simulink subsystem "MultibodySuspensionSSC"  (R2025a)
settings: Solver=VariableStepAuto  StartTime=0.0  StopTime=10.0  RelTol=1e-3
undefined symbols (not defined in the file): EnvGrvty, FrntRef, LAc, LAf, LAr, PlntVehDstCGFrntAxl, PlntVehDstCGRearAxl, PlntVehMass, PlntVehMultiBody, PlntVehMultiBodyGeom, RearRef, StrRodFL, StrRodFR, StrRodRL, StrRodRR, UAc, UAf, UAr, WheelFL, WheelFR, WheelRL, WheelRR, X, Y, Z
libraries: sm_lib x450, fl_lib x96, nesl_utility x64, sdl_lib x8
(part 3 of 17)

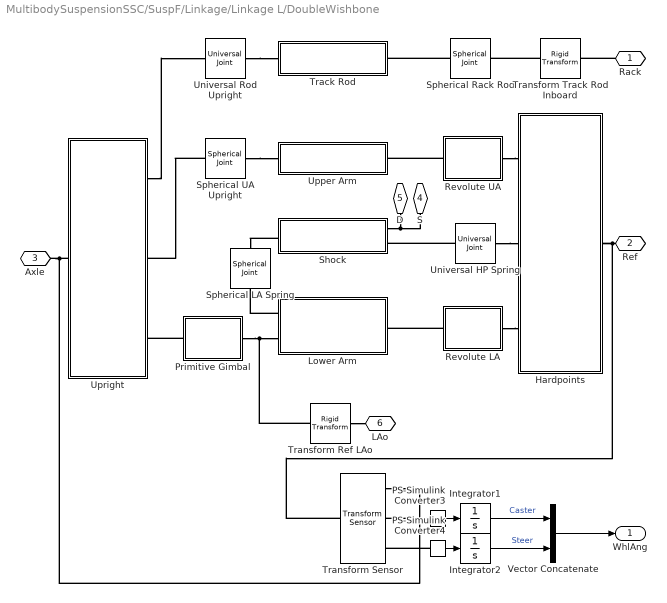
== system MultibodySuspensionSSC/SuspF/Linkage/Linkage L/DoubleWishbone ==
  Hardpoints : Subsystem  mask(Hardpoints, Subframe and Chassis){popup_leftRight=Left, hp_in_f_ua=hp_in_f_ua, hp_in_r_ua=hp_in_r_ua, hp_in_f_la=hp_in_f_la, hp_in_r_la=hp_in_r_la, hp_spr_top=hp_spr_top, clr_hp=clr_hp, opc_hp=opc_hp, size_hp=size_hp}
      mask prompts: popup_leftRight "Left/Right"; hp_in_f_ua "Upper Arm Front [xyz] (m)"; hp_in_r_ua "Upper Arm Rear [xyz] (m)"; hp_in_f_la "Lower Arm Front [xyz] (m)"; hp_in_r_la "Lower Arm Rear [xyz] (m)"; hp_spr_top "Spring [xyz] (m)"
      mask help: Hardpoints for linkage connection points to chassis. Defined relative to an axle reference point.
      mask init:
      | % Set parameter for mirroring (+y or -y)
      | if(popup_leftRight == 1)
      |     rhs_susp = 1;    
      | elseif(popup_leftRight == 2)
      |     rhs_susp = -1;
      | end
      | 
      | rhs_hp = [1 rhs_susp 1];
      | 
      | % Calculate lengths and displacments
      | %len_la_f2r = norm(hp_in_f_la-hp_in_r_la);
      | %len_ua_f2r = norm(hp_in_f_ua-hp_in_r_ua);
      | 
      | % Calculate angle between arm-to-chassis attachment axis
      | % and outboard to inboard front, outboard to inboard rear.
      | % Used to orient z-axis of hardpoint frames along vector 
      | % from inboard points to outboard point.
      | % Angles calculated in World Frame
      | %angle_la_f2r_yaw   =  atan2d(hp_in_f_la(2)-hp_in_r_la(2),hp_in_f_la(1)-hp_in_r_la(1));
      | %angle_la_f2r_pitch = -asind((hp_in_f_la(3)-hp_in_r_la(3))/len_la_f2r);
      | 
      | %angle_ua_f2r_yaw   =  atan2d(hp_in_f_ua(2)-hp_in_r_ua(2),hp_in_f_ua(1)-hp_in_r_ua(1));
      | %angle_ua_f2r_pitch = -asind((hp_in_f_ua(3)-hp_in_r_ua(3))/len_ua_f2r);
      mask TypeOptions popup_leftRight: Left | Right
      mask TypeOptions clr_hp: Subsystem/Vis HP LAf/GraphicDiffuseColor | Vis HP LAr/GraphicDiffuseColor | Vis HP Spring/GraphicDiffuseColor | Vis HP UAf/GraphicDiffuseColor | Vis HP UAr/GraphicDiffuseColor
      mask TypeOptions opc_hp: Subsystem/Vis HP LAf/GraphicOpacity | Vis HP LAr/GraphicOpacity | Vis HP Spring/GraphicOpacity | Vis HP UAf/GraphicOpacity | Vis HP UAr/GraphicOpacity
      mask DialogControl cont_hp Prompt: Hardpoints
      mask DialogControl cont_vis_hp Prompt: Visualization
      mask DialogControl text_clr_hp Prompt: Color [RGB]
      mask DialogControl text_opc_hp Prompt: Opac. (0-1)
      mask DialogControl text_size_hp Prompt: Size (m)
      mask DialogControl text_hp Prompt: Hardpoints
  Integrator1 : Integrator
  Integrator2 : Integrator
  Lower Arm : Subsystem  mask(Lower Arm (Wishbone)){popup_leftRight=Left, hp_in_f=hp_in_f_la, hp_in_r=hp_in_r_la, hp_out=hp_out_la, hp_spr=hp_spr_bot, la_mass=la_mass, clr_la=clr_la, opc_la=opc_la, radius_la=radius_la}
      mask prompts: popup_leftRight "Left/Right"; hp_in_f "Inboard Front [xyz] (m)"; hp_in_r "Inboard Rear [xyz] (m)"; hp_out "Outboard [xyz] (m)"; hp_spr "Spring [xyz] (m)"; la_mass "Mass (kg)"; clr_la "Color [RGB]"; opc_la "Opacity (0-1)"; radius_la "Radius (m)"
      mask help: This subsystem models the lower arm of a wishbone suspension. It can be configured to have one or two attachment points to the chassis. There are connections to the upright and spring.
      mask init:
      | % Set parameter for mirroring (+y or -y)
      | if(popup_leftRight == 1)
      |     rhs_susp = 1;
      | elseif(popup_leftRight == 2)
      |     rhs_susp = -1;
      | end
      | 
      | rhs_hp = [1 rhs_susp 1];
      | 
      | % Calculate lengths and displacments
      | %%%len_front = norm(hp_in_f-hp_out);
      | %%%len_rear  = norm(hp_in_r-hp_out);
      | %%%dist_f2r  = norm(hp_in_f-hp_in_r);
      | 
      | % Vector from outboard hardpoint to spring attachment
      | % Expressed in *World* coordinates
      | %%%xyz_out2spr  = hp_spr-hp_out;
      | 
      | % Calculate angles to align z-axis of arm frames
      | % along vector from inboard points to outboard point
      | % - WORLD FRAME
      | %angle_f2r_pitch = -atan2d(hp_in_f(3)-hp_in_r(3),hp_in_f(1)-hp_in_r(1));
      | %angle_f2r_yaw = atan2d(hp_in_f(2)-hp_in_r(2),hp_in_f(1)-hp_in_r(1));
      | 
      | % Calculate angle between arm-to-chassis attachment axis
      | % and outboard to inboard front, outboard to inboard rear
      | % about axis normal to the arm.
      | % Used to orient z-axis of arm frames along vector 
      | % from inboard points to outboard point
      | %%%angle_f2r_f2out = sm_math_angle_3hp(hp_in_r, hp_in_f, hp_out);
      | %%%angle_r2f_r2out = sm_math_angle_3hp(hp_in_f, hp_in_r, hp_out);
      | 
      | % Obtain angles to reorient frame at outboard hardpoint to global frame
      | % so that outboard to spring attachment calculation can be used
      | % WORLD FRAME - not used
      | %angle_f2r_pitch = sm_math_angle_3hp(hp_in_f.*[1 0 1], hp_in_r.*[1 0 1], [hp_in_f(1) 0 hp_in_r(3)])*sign(hp_in_r(3)-hp_in_f(3))
      | %angle_f2r_yaw = sm_math_angle_3hp(hp_in_f.*[1 1 0], hp_in_r.*[1 1 0], [hp_in_f(1) hp_in_r(2) 0])*sign(hp_in_r(2)-hp_in_f(2))
      | 
      | % Obtain angles to reorient frame at outboard hardpoint to global frame
      | % so that outboard to spring vector in world frame (xyz_out2spr)can be
      | % used. Angles in arm reference frame. 
      | % Same calculation as in hardpoints subsystem.
      | %angle_la_f2r_pitch = -atan2d(hp_in_f(3)-hp_in_r(3),hp_in_f(1)-hp_in_r(1));
      | %angle_la_f2r_yaw   =  atan2d(hp_in_f(2)-hp_in_r(2),hp_in_f(1)-hp_in_r(1));
      | %%%angle_la_f2r_yaw   =  atan2d(hp_in_f(2)-hp_in_r(2),hp_in_f(1)-hp_in_r(1));
      | %%%angle_la_f2r_pitch = -asind((hp_in_f(3)-hp_in_r(3))/dist_f2r);
      | 
      | % -- Calculate rotation of lower arm about joint axis --
      | % Obtain shortest distance from outboard to inboard hardpoint axis
      | % Hypotenuse of triangle for obtaining rotation of arm
      | %%%dist_out2fraxis=len_front*sind(angle_f2r_f2out);
      | 
      | % - Obtain vertical distance of triangle for obtaining rotation of arm
      | % Rotate Inboard Front -> Inboard Rear vector       (r2f)
      | % and Inboard Front -> Outboard vector by yaw angle (r2o)
      | %%%r2f_new = sm_math_rotbasic(hp_in_f'-hp_in_r',-angle_la_f2r_yaw,'z');
      | %%%r2o_new = sm_math_rotbasic(hp_out'-hp_in_r',-angle_la_f2r_yaw,'z');
      | 
      | % Rotate these vectors by pitch angle 
      | %%%r2f_wld = sm_math_rotbasic(r2f_new,-angle_la_f2r_pitch,'y');
      | %%%r2o_wld = sm_math_rotbasic(r2o_new,-angle_la_f2r_pitch,'y');
      | 
      | % Height for angle calculation
      | % After two rotations, can look at z-axis components
      | %%%xangle_height = r2f_wld(3)-r2o_wld(3);
      | 
      | % Calculate angle about f-r axis
      | %%%angle_la_f2raxis = asind(xangle_height/dist_out2fraxis);
      | 
      | % Need additional point to figure out angle with respect to global x-axis
      | % WORLD - Not used
      | %dxpcnt_outfraxis = (hp_out(1)-hp_in_r(1))/(hp_in_f(1)-hp_in_r(1));
      | %hp_rollcalc = hp_in_r+(hp_in_f-hp_in_r)*dxpcnt_outfraxis;
      | %angle_outfr_roll = -sm_math_angle_3hp(hp_rollcalc.*[0 1 1], hp_out.*[0 1 1], [0 hp_rollcalc(2) hp_out(3)])
      | %angle_outfr_roll = -atan2d(hp_out(3)-hp_rollcalc(3),hp_out(2)-hp_rollcalc(2));
      mask Help: web ('sm_car_lower_arm_help.html')
      mask TypeOptions popup_leftRight: Left | Right
      mask TypeOptions clr_la: Arm F/clr_solid | Arm R/clr_solid | Arm Spring/clr_solid
      mask TypeOptions opc_la: Arm F/opc_solid | Arm R/opc_solid | Arm Spring/opc_solid
      mask TypeOptions radius_la: Arm F/rad_solid | Arm R/rad_solid | Arm Spring/rad_solid
      mask DialogControl cont_ua Prompt: LA
      mask DialogControl cont_vis_la Prompt: Visualization
  PS-Simulink Converter3 : nesl_utility/PS-Simulink Converter  PhysicalDomain=network_engine_domain  SubClassName=ps_output  LeftPortType=input  RightPortType=output  PseudoPeriodic=off  Frequencies=[]  VectorFormat=inherit  Unit=inherit  AffineConversion=off
  PS-Simulink Converter4 : nesl_utility/PS-Simulink Converter  PhysicalDomain=network_engine_domain  SubClassName=ps_output  LeftPortType=input  RightPortType=output  PseudoPeriodic=off  Frequencies=[]  VectorFormat=inherit  Unit=inherit  AffineConversion=off
  Primitive Gimbal : Subsystem
      settings: LibrarySourceBlock=sm_car_4post_lib/Suspension and Steering/Linkage/Linkage L/DoubleWishbone/Primitive Gimbal
  Revolute LA : Subsystem  VariantControl=Rigid_1Rev
  Revolute UA : Subsystem  VariantControl=Rigid_1Rev
  Shock : Subsystem  mask(Shock){shock_pist_mass=shock_pist_mass, shock_cyl_mass=shock_cyl_mass, hp_spr_top=hp_spr_top, hp_spr_bot=hp_spr_bot, up_lim_bumpstop=up_lim_bumpstop, low_lim_bumpstop=low_lim_bumpstop, clr_conn_shock=clr_conn_shock, opc_conn_shock=opc_conn_shock, size_conn_shock=size_conn_shock, clr_shock_cyl=clr_shock_cyl, opc_shock_cyl=opc_shock_cyl, radius_shock_cyl=radius_shock_cyl, clr_shock_piston=clr_shock_piston, opc_shock_piston=opc_shock_piston, clr_shock_bumpstop=clr_shock_bumpstop, opc_shock_bumpstop=opc_shock_bumpstop, deadvol_len_shock_cyl=deadvol_len_shock_cyl, piston_len_shock=piston_len_shock, cyl_cap_len_shock=cyl_cap_len_shock, bumpstop_len_shock=bumpstop_len_shock}
      mask prompts: shock_pist_mass "Piston Mass (kg)"; shock_cyl_mass "Cylinder Mass (kg)"; hp_spr_top "Spring Top [xyz] (m)"; hp_spr_bot "Spring Bottom [xyz] (m)"; up_lim_bumpstop "Upper Limit Bumpstop (m)"; low_lim_bumpstop "Lower Limit Bumpstop (m)"; deadvol_len_shock_cyl "Dead Volume Height (m)"; piston_len_shock "Piston Length (m)"; cyl_cap_len_shock "Cylinder Cap Length (m)"; bumpstop_len_shock "Bumpstop Length (m)"
      mask help: Mechanical parts and joint modeling shock absorber.
      mask init:
      | init_spr_len = norm(hp_spr_top-hp_spr_bot);
      | 
      | rod_length = init_spr_len-deadvol_len_shock_cyl-cyl_cap_len_shock-abs(low_lim_bumpstop);
      | 
      | bumpstop_xc_rev = [0 0; 0.5 0; 0.7 1; 0 1].*[radius_shock_cyl bumpstop_len_shock];
      | 
      | cyl_wall_length = piston_len_shock+abs(low_lim_bumpstop)+abs(up_lim_bumpstop)+deadvol_len_shock_cyl;
      mask TypeOptions shock_pist_mass: Piston/Rod/Mass
      mask TypeOptions shock_cyl_mass: Cylinder/Wall/Mass
      mask TypeOptions clr_conn_shock:
      | Vis
      | Spring
      | LA/GraphicDiffuseColor | Vis
      | Spring
      | HP/GraphicDiffuseColor
      mask TypeOptions opc_conn_shock:
      | Vis
      | Spring
      | LA/GraphicOpacity | Vis
      | Spring
      | HP/GraphicOpacity
      mask TypeOptions clr_shock_cyl: Cylinder/Cap Bottom/GraphicDiffuseColor | Cylinder/Cap Top/GraphicDiffuseColor | Cylinder/Wall/GraphicDiffuseColor
      mask TypeOptions clr_shock_piston: Piston/Cap/GraphicDiffuseColor | Piston/Piston/GraphicDiffuseColor | Piston/Rod/GraphicDiffuseColor
      mask TypeOptions opc_shock_piston: Piston/Cap/GraphicOpacity | Piston/Piston/GraphicOpacity | Piston/Rod/GraphicOpacity
      mask TypeOptions clr_shock_bumpstop: Piston/Bumpstop/GraphicDiffuseColor
      mask TypeOptions opc_shock_bumpstop: Piston/Bumpstop/GraphicOpacity
      mask DialogControl cont_shock Prompt: Shock
      mask DialogControl cont_vis_shock Prompt: Visualization
      mask DialogControl text_clr_shock Prompt: Color  [RGB]
      mask DialogControl text_opc_shock Prompt: Opac. (0-1)
      mask DialogControl text_size_shock Prompt: Size (m)
      mask DialogControl text_conn_shock Prompt: Connections
      mask DialogControl text_shock_cyl Prompt: Cylinder
      mask DialogControl text_shock_piston Prompt: Piston
      mask DialogControl text_piston_radius Prompt: <cylinder radius>
      mask DialogControl text_shock_bumpstop Prompt: Bumpstop
      mask DialogControl text_bumpstop_radius Prompt: <cylinder radius>
  Spherical LA Spring : sm_lib/Joints/Spherical Joint  JointMode=Normal  CompositeWrenchDir=FollowerOnBase  CompositeWrenchFrame=BaseFrame  SenseConstraintForce=off  SenseConstraintTorque=off  SenseTotalForce=off  SenseTotalTorque=off  PositionTargetSpecify=off  PositionTargetPriority=High  PositionTargetRotationMethod=None  PositionTargetFollAlignAxisA=+X  PositionTargetBaseAlignAxisA=+Y  PositionTargetFollAlignAxisB=+Y  PositionTargetBaseAlignAxisB=+Z  PositionTargetRotationStandardAxis=+Z  PositionTargetRotationAngle=0.0  PositionTargetRotationAngleUnits=deg  PositionTargetRotationArbitraryAxis=[0 0 1]  PositionTargetRotationSequenceAxes=FollowerAxes  PositionTargetRotationSequence=XYX  PositionTargetRotationSequenceAngles=[0 0 0]  PositionTargetRotationSequenceAnglesUnits=deg  PositionTargetRotationMatrix=[1 0 0; 0 1 0; 0 0 1]  PositionTargetQuaternion=[1 0 0 0]  VelocityTargetSpecify=off  VelocityTargetPriority=High  VelocityTargetValue=[0 0 0]  VelocityTargetValueUnits=deg/s  VelocityTargetInFollowerFrame=on  EqPosRotationMethod=None  EqPosFollAlignAxisA=+X  EqPosBaseAlignAxisA=+Y  EqPosFollAlignAxisB=+Y  EqPosBaseAlignAxisB=+Z  EqPosRotationStandardAxis=+Z  EqPosRotationAngle=0.0  EqPosRotationAngleUnits=deg  EqPosRotationArbitraryAxis=[0 0 1]  EqPosRotationSequenceAxes=FollowerAxes  EqPosRotationSequence=XYX  EqPosRotationSequenceAngles=[0 0 0]  EqPosRotationSequenceAnglesUnits=deg  EqPosRotationMatrix=[1 0 0; 0 1 0; 0 0 1]  EqPosQuaternion=[1 0 0 0]  SpringStiffness=0  SpringStiffnessUnits=N*m/deg  DampingCoefficient=0  DampingCoefficientUnits=N*m/(deg/s)  LowerLimitSpecify=off  LowerLimitBound=15  LowerLimitBoundUnits=deg  LowerLimitStiffness=1e4  LowerLimitStiffnessUnits=N*m/deg  LowerLimitDamping=10  LowerLimitDampingUnits=N*m/(deg/s)  LowerLimitTransitionRegionWidth=0.1  LowerLimitTransitionRegionWidthUnits=deg  UpperLimitSpecify=off  UpperLimitBound=45  UpperLimitBoundUnits=deg  UpperLimitStiffness=1e4  UpperLimitStiffnessUnits=N*m/deg  UpperLimitDamping=10  UpperLimitDampingUnits=N*m/(deg/s)  UpperLimitTransitionRegionWidth=0.1  UpperLimitTransitionRegionWidthUnits=deg  TorqueActuationMode=NoTorque  ActuateTorqueX=off  ActuateTorqueY=off  ActuateTorqueZ=off  ActuateTorque=off  ActuationFrame=BaseFrame  SensePosition=off  SenseVelocityX=off  SenseVelocityY=off  SenseVelocityZ=off  SenseVelocity=off  SenseAccelerationX=off  SenseAccelerationY=off  SenseAccelerationZ=off  SenseAcceleration=off  SenseLowerLimitTorqueMag=off  SenseUpperLimitTorqueMag=off  SensingFrame=BaseFrame
      settings: LibrarySourceBlock=|
      | sm_car_4post_lib/Suspension and Steering/Linkage/Linkage L/DoubleWishbone/Spherical
      | LA Spring
  Spherical Rack Rod : sm_lib/Joints/Spherical Joint  JointMode=Normal  CompositeWrenchDir=FollowerOnBase  CompositeWrenchFrame=BaseFrame  SenseConstraintForce=off  SenseConstraintTorque=off  SenseTotalForce=off  SenseTotalTorque=off  PositionTargetSpecify=off  PositionTargetPriority=High  PositionTargetRotationMethod=None  PositionTargetFollAlignAxisA=+X  PositionTargetBaseAlignAxisA=+Y  PositionTargetFollAlignAxisB=+Y  PositionTargetBaseAlignAxisB=+Z  PositionTargetRotationStandardAxis=+Z  PositionTargetRotationAngle=0.0  PositionTargetRotationAngleUnits=deg  PositionTargetRotationArbitraryAxis=[0 0 1]  PositionTargetRotationSequenceAxes=FollowerAxes  PositionTargetRotationSequence=XYX  PositionTargetRotationSequenceAngles=[0 0 0]  PositionTargetRotationSequenceAnglesUnits=deg  PositionTargetRotationMatrix=[1 0 0; 0 1 0; 0 0 1]  PositionTargetQuaternion=[1 0 0 0]  VelocityTargetSpecify=off  VelocityTargetPriority=High  VelocityTargetValue=[0 0 0]  VelocityTargetValueUnits=deg/s  VelocityTargetInFollowerFrame=on  EqPosRotationMethod=None  EqPosFollAlignAxisA=+X  EqPosBaseAlignAxisA=+Y  EqPosFollAlignAxisB=+Y  EqPosBaseAlignAxisB=+Z  EqPosRotationStandardAxis=+Z  EqPosRotationAngle=0.0  EqPosRotationAngleUnits=deg  EqPosRotationArbitraryAxis=[0 0 1]  EqPosRotationSequenceAxes=FollowerAxes  EqPosRotationSequence=XYX  EqPosRotationSequenceAngles=[0 0 0]  EqPosRotationSequenceAnglesUnits=deg  EqPosRotationMatrix=[1 0 0; 0 1 0; 0 0 1]  EqPosQuaternion=[1 0 0 0]  SpringStiffness=0  SpringStiffnessUnits=N*m/deg  DampingCoefficient=0  DampingCoefficientUnits=N*m/(deg/s)  LowerLimitSpecify=off  LowerLimitBound=15  LowerLimitBoundUnits=deg  LowerLimitStiffness=1e4  LowerLimitStiffnessUnits=N*m/deg  LowerLimitDamping=10  LowerLimitDampingUnits=N*m/(deg/s)  LowerLimitTransitionRegionWidth=0.1  LowerLimitTransitionRegionWidthUnits=deg  UpperLimitSpecify=off  UpperLimitBound=45  UpperLimitBoundUnits=deg  UpperLimitStiffness=1e4  UpperLimitStiffnessUnits=N*m/deg  UpperLimitDamping=10  UpperLimitDampingUnits=N*m/(deg/s)  UpperLimitTransitionRegionWidth=0.1  UpperLimitTransitionRegionWidthUnits=deg  TorqueActuationMode=NoTorque  ActuateTorqueX=off  ActuateTorqueY=off  ActuateTorqueZ=off  ActuateTorque=off  ActuationFrame=BaseFrame  SensePosition=off  SenseVelocityX=off  SenseVelocityY=off  SenseVelocityZ=off  SenseVelocity=off  SenseAccelerationX=off  SenseAccelerationY=off  SenseAccelerationZ=off  SenseAcceleration=off  SenseLowerLimitTorqueMag=off  SenseUpperLimitTorqueMag=off  SensingFrame=BaseFrame
      settings: LibrarySourceBlock=|
      | sm_car_4post_lib/Suspension and Steering/Linkage/Linkage L/DoubleWishbone/Spherical
      | Rack Rod
  Spherical UA Upright : sm_lib/Joints/Spherical Joint  JointMode=Normal  CompositeWrenchDir=FollowerOnBase  CompositeWrenchFrame=BaseFrame  SenseConstraintForce=off  SenseConstraintTorque=off  SenseTotalForce=off  SenseTotalTorque=off  PositionTargetSpecify=on  PositionTargetPriority=High  PositionTargetRotationMethod=StandardAxis  PositionTargetFollAlignAxisA=+X  PositionTargetBaseAlignAxisA=+Y  PositionTargetFollAlignAxisB=+Y  PositionTargetBaseAlignAxisB=+Z  PositionTargetRotationStandardAxis=+Z  PositionTargetRotationAngle=0.0  PositionTargetRotationAngleUnits=deg  PositionTargetRotationArbitraryAxis=[0 0 1]  PositionTargetRotationSequenceAxes=FollowerAxes  PositionTargetRotationSequence=XYX  PositionTargetRotationSequenceAngles=[0 0 0]  PositionTargetRotationSequenceAnglesUnits=deg  PositionTargetRotationMatrix=[1 0 0; 0 1 0; 0 0 1]  PositionTargetQuaternion=[1 0 0 0]  VelocityTargetSpecify=off  VelocityTargetPriority=High  VelocityTargetValue=[0 0 0]  VelocityTargetValueUnits=deg/s  VelocityTargetInFollowerFrame=on  EqPosRotationMethod=None  EqPosFollAlignAxisA=+X  EqPosBaseAlignAxisA=+Y  EqPosFollAlignAxisB=+Y  EqPosBaseAlignAxisB=+Z  EqPosRotationStandardAxis=+Z  EqPosRotationAngle=0.0  EqPosRotationAngleUnits=deg  EqPosRotationArbitraryAxis=[0 0 1]  EqPosRotationSequenceAxes=FollowerAxes  EqPosRotationSequence=XYX  EqPosRotationSequenceAngles=[0 0 0]  EqPosRotationSequenceAnglesUnits=deg  EqPosRotationMatrix=[1 0 0; 0 1 0; 0 0 1]  EqPosQuaternion=[1 0 0 0]  SpringStiffness=0  SpringStiffnessUnits=N*m/deg  DampingCoefficient=0  DampingCoefficientUnits=N*m/(deg/s)  LowerLimitSpecify=off  LowerLimitBound=15  LowerLimitBoundUnits=deg  LowerLimitStiffness=1e4  LowerLimitStiffnessUnits=N*m/deg  LowerLimitDamping=10  LowerLimitDampingUnits=N*m/(deg/s)  LowerLimitTransitionRegionWidth=0.1  LowerLimitTransitionRegionWidthUnits=deg  UpperLimitSpecify=off  UpperLimitBound=45  UpperLimitBoundUnits=deg  UpperLimitStiffness=1e4  UpperLimitStiffnessUnits=N*m/deg  UpperLimitDamping=10  UpperLimitDampingUnits=N*m/(deg/s)  UpperLimitTransitionRegionWidth=0.1  UpperLimitTransitionRegionWidthUnits=deg  TorqueActuationMode=NoTorque  ActuateTorqueX=off  ActuateTorqueY=off  ActuateTorqueZ=off  ActuateTorque=off  ActuationFrame=BaseFrame  SensePosition=off  SenseVelocityX=off  SenseVelocityY=off  SenseVelocityZ=off  SenseVelocity=off  SenseAccelerationX=off  SenseAccelerationY=off  SenseAccelerationZ=off  SenseAcceleration=off  SenseLowerLimitTorqueMag=off  SenseUpperLimitTorqueMag=off  SensingFrame=BaseFrame
      settings: LibrarySourceBlock=|
      | sm_car_4post_lib/Suspension and Steering/Linkage/Linkage L/DoubleWishbone/Spherical
      | UA Upright
  Track Rod : Subsystem  VariantControl=Steer  mask{popup_leftRight=Left, hp_in=hp_in_rod, hp_out=hp_upr_rod, rod_mass=rod_mass, clr_conn_rod=clr_conn_rod, opc_conn_rod=opc_conn_rod, size_conn_rod=size_conn_rod, clr_rod=clr_rod, opc_rod=opc_rod, radius_rod=radius_rod}
      mask prompts: popup_leftRight "Left/Right"; hp_in "Inboard [xyz] (m)"; hp_out "Outboard [xyz] (m)"; rod_mass "Mass (kg)"; clr_rod "Color [RGB]"; opc_rod "Opacity (0-1)"; radius_rod "Radius (m)"
      mask init:
      | if(popup_leftRight == 1)
      |     rhs_rod = 1;
      | elseif(popup_leftRight == 2)
      |     rhs_rod = -1;
      | end
      | 
      | % Calculate lengths
      | %%%rod_len = norm(hp_out-hp_in);
      mask TypeOptions popup_leftRight: Left | Right
      mask TypeOptions rod_mass: Rod/Mass
      mask TypeOptions clr_conn_rod:
      | Vis
      | Upright
      | Steer/GraphicDiffuseColor | Vis
      | Rack
      | Rod/GraphicDiffuseColor
      mask TypeOptions opc_conn_rod:
      | Vis
      | Upright
      | Steer/GraphicOpacity | Vis
      | Rack
      | Rod/GraphicOpacity
      mask TypeOptions clr_rod: Rod/clr_solid
      mask TypeOptions opc_rod: Rod/opc_solid
      mask TypeOptions radius_rod: Rod/rad_solid
      mask DialogControl cont_rod Prompt: Rod
      mask DialogControl grp_rod Prompt: Rod
      mask DialogControl cont_vis_rod Prompt: Visualization
      mask DialogControl text_clr_rod Prompt: Color [RGB]
      mask DialogControl text_opc_rod Prompt: Opac. (0-1)
      mask DialogControl text_size_rod Prompt: Size (m)
      mask DialogControl text_conn_rod Prompt: Connections
      mask DialogControl text_rod_rod Prompt: Rod
  Transform Ref LAo : sm_lib/Frames and Transforms/Rigid Transform  RotationMethod=None  FollAlignAxisA=+X  BaseAlignAxisA=+Y  FollAlignAxisB=+Y  BaseAlignAxisB=+Z  RotationStandardAxis=+Z  RotationAngle=0.0  RotationAngleUnits=deg  RotationArbitraryAxis=[0 0 1]  RotationSequenceAxes=FollowerAxes  RotationSequence=XYX  RotationSequenceAngles=[0 0 0]  RotationSequenceAnglesUnits=deg  RotationMatrix=[1 0 0; 0 1 0; 0 0 1]  Quaternion=[1 0 0 0]  TranslationMethod=Cartesian  TranslationCartesianOffset=hp_out_la.*[1 rhs_susp 1]  TranslationCartesianOffsetUnits=m  TranslationStandardAxis=+Z  TranslationStandardOffset=0  TranslationStandardOffsetUnits=m  TranslationROffset=0  TranslationROffsetUnits=m  TranslationThetaOffset=0  TranslationThetaOffsetUnits=deg  TranslationZOffset=0  TranslationZOffsetUnits=m
  Transform Sensor : sm_lib/Frames and Transforms/Transform Sensor  MeasurementFrame=NonRotatingBase  RotationSequence=XYX  SenseAngle=off  SenseAxis=off  SenseQ=off  SenseR=off  SenseRotationSequence=off  SenseOmegaX=off  SenseOmegaY=on  SenseOmegaZ=on  SenseOmega=off  SenseQDot=off  SenseRDot=off  SenseRotationSequenceDot=off  SenseAlphaX=off  SenseAlphaY=off  SenseAlphaZ=off  SenseAlpha=off  SenseQDDot=off  SenseRDDot=off  SenseX=off  SenseY=off  SenseZ=off  SenseXYZ=off  SenseRad=off  SenseAzim=off  SenseDist=off  SenseInc=off  SenseXDot=off  SenseYDot=off  SenseZDot=off  SenseXYZDot=off  SenseRadDot=off  SenseAzimDot=off  SenseDistDot=off  SenseIncDot=off  SenseXDDot=off  SenseYDDot=off  SenseZDDot=off  SenseXYZDDot=off  SenseRadDDot=off  SenseAzimDDot=off  SenseDistDDot=off  SenseIncDDot=off
  Transform Track Rod Inboard : sm_lib/Frames and Transforms/Rigid Transform  RotationMethod=None  FollAlignAxisA=+X  BaseAlignAxisA=+Y  FollAlignAxisB=+Y  BaseAlignAxisB=+Z  RotationStandardAxis=+Z  RotationAngle=0.0  RotationAngleUnits=deg  RotationArbitraryAxis=[0 0 1]  RotationSequenceAxes=FollowerAxes  RotationSequence=XYX  RotationSequenceAngles=[0 0 0]  RotationSequenceAnglesUnits=deg  RotationMatrix=[1 0 0; 0 1 0; 0 0 1]  Quaternion=[1 0 0 0]  TranslationMethod=Cartesian  TranslationCartesianOffset=hp_in_rod.*[1 rhs_susp 1]  TranslationCartesianOffsetUnits=m  TranslationStandardAxis=+Z  TranslationStandardOffset=0  TranslationStandardOffsetUnits=m  TranslationROffset=0  TranslationROffsetUnits=m  TranslationThetaOffset=0  TranslationThetaOffsetUnits=deg  TranslationZOffset=0  TranslationZOffsetUnits=m
      settings: LibrarySourceBlock=|
      | sm_car_4post_lib/Suspension and Steering/Linkage/Linkage L/DoubleWishbone/Transform
      | Track Rod Inboard
  Universal HP Spring : sm_lib/Joints/Universal Joint  JointMode=Normal  CompositeWrenchDir=FollowerOnBase  CompositeWrenchFrame=BaseFrame  SenseConstraintForce=off  SenseConstraintTorque=off  SenseTotalForce=off  SenseTotalTorque=off  RxPositionTargetSpecify=off  RxPositionTargetPriority=High  RxPositionTargetValue=0  RxPositionTargetValueUnits=deg  RxVelocityTargetSpecify=off  RxVelocityTargetPriority=High  RxVelocityTargetValue=0  RxVelocityTargetValueUnits=deg/s  RxEquilibriumPosition=0  RxEquilibriumPositionUnits=deg  RxSpringStiffness=0  RxSpringStiffnessUnits=N*m/deg  RxDampingCoefficient=0  RxDampingCoefficientUnits=N*m/(deg/s)  RxLowerLimitSpecify=off  RxLowerLimitBound=-90  RxLowerLimitBoundUnits=deg  RxLowerLimitStiffness=1e4  RxLowerLimitStiffnessUnits=N*m/deg  RxLowerLimitDamping=10  RxLowerLimitDampingUnits=N*m/(deg/s)  RxLowerLimitTransitionRegionWidth=0.1  RxLowerLimitTransitionRegionWidthUnits=deg  RxUpperLimitSpecify=off  RxUpperLimitBound=90  RxUpperLimitBoundUnits=deg  RxUpperLimitStiffness=1e4  RxUpperLimitStiffnessUnits=N*m/deg  RxUpperLimitDamping=10  RxUpperLimitDampingUnits=N*m/(deg/s)  RxUpperLimitTransitionRegionWidth=0.1  RxUpperLimitTransitionRegionWidthUnits=deg  RxTorqueActuationMode=NoTorque  RxMotionActuationMode=ComputedMotion  RxSensePosition=off  RxSenseVelocity=off  RxSenseAcceleration=off  RxSenseTorqueForce=off  RxSenseLowerLimitTorqueForce=off  RxSenseUpperLimitTorqueForce=off  RyPositionTargetSpecify=off  RyPositionTargetPriority=High  RyPositionTargetValue=0  RyPositionTargetValueUnits=deg  RyVelocityTargetSpecify=off  RyVelocityTargetPriority=High  RyVelocityTargetValue=0  RyVelocityTargetValueUnits=deg/s  RyEquilibriumPosition=0  RyEquilibriumPositionUnits=deg  RySpringStiffness=0  RySpringStiffnessUnits=N*m/deg  RyDampingCoefficient=0  RyDampingCoefficientUnits=N*m/(deg/s)  RyLowerLimitSpecify=off  RyLowerLimitBound=-90  RyLowerLimitBoundUnits=deg  RyLowerLimitStiffness=1e4  RyLowerLimitStiffnessUnits=N*m/deg  RyLowerLimitDamping=10  RyLowerLimitDampingUnits=N*m/(deg/s)  RyLowerLimitTransitionRegionWidth=0.1  RyLowerLimitTransitionRegionWidthUnits=deg  RyUpperLimitSpecify=off  RyUpperLimitBound=90  RyUpperLimitBoundUnits=deg  RyUpperLimitStiffness=1e4  RyUpperLimitStiffnessUnits=N*m/deg  RyUpperLimitDamping=10  RyUpperLimitDampingUnits=N*m/(deg/s)  RyUpperLimitTransitionRegionWidth=0.1  RyUpperLimitTransitionRegionWidthUnits=deg  RyTorqueActuationMode=NoTorque  RyMotionActuationMode=ComputedMotion  RySensePosition=off  RySenseVelocity=off  RySenseAcceleration=off  RySenseTorqueForce=off  RySenseLowerLimitTorqueForce=off  RySenseUpperLimitTorqueForce=off
      settings: LibrarySourceBlock=|
      | sm_car_4post_lib/Suspension and Steering/Linkage/Linkage L/DoubleWishbone/Universal
      | HP Spring
  Universal Rod Upright : sm_lib/Joints/Universal Joint  JointMode=Normal  CompositeWrenchDir=FollowerOnBase  CompositeWrenchFrame=BaseFrame  SenseConstraintForce=off  SenseConstraintTorque=off  SenseTotalForce=off  SenseTotalTorque=off  RxPositionTargetSpecify=off  RxPositionTargetPriority=Low  RxPositionTargetValue=0  RxPositionTargetValueUnits=deg  RxVelocityTargetSpecify=off  RxVelocityTargetPriority=High  RxVelocityTargetValue=0  RxVelocityTargetValueUnits=deg/s  RxEquilibriumPosition=0  RxEquilibriumPositionUnits=deg  RxSpringStiffness=0  RxSpringStiffnessUnits=N*m/deg  RxDampingCoefficient=0  RxDampingCoefficientUnits=N*m/(deg/s)  RxLowerLimitSpecify=off  RxLowerLimitBound=-90  RxLowerLimitBoundUnits=deg  RxLowerLimitStiffness=1e4  RxLowerLimitStiffnessUnits=N*m/deg  RxLowerLimitDamping=10  RxLowerLimitDampingUnits=N*m/(deg/s)  RxLowerLimitTransitionRegionWidth=0.1  RxLowerLimitTransitionRegionWidthUnits=deg  RxUpperLimitSpecify=off  RxUpperLimitBound=90  RxUpperLimitBoundUnits=deg  RxUpperLimitStiffness=1e4  RxUpperLimitStiffnessUnits=N*m/deg  RxUpperLimitDamping=10  RxUpperLimitDampingUnits=N*m/(deg/s)  RxUpperLimitTransitionRegionWidth=0.1  RxUpperLimitTransitionRegionWidthUnits=deg  RxTorqueActuationMode=NoTorque  RxMotionActuationMode=ComputedMotion  RxSensePosition=off  RxSenseVelocity=off  RxSenseAcceleration=off  RxSenseTorqueForce=off  RxSenseLowerLimitTorqueForce=off  RxSenseUpperLimitTorqueForce=off  RyPositionTargetSpecify=off  RyPositionTargetPriority=High  RyPositionTargetValue=0  RyPositionTargetValueUnits=deg  RyVelocityTargetSpecify=off  RyVelocityTargetPriority=High  RyVelocityTargetValue=0  RyVelocityTargetValueUnits=deg/s  RyEquilibriumPosition=0  RyEquilibriumPositionUnits=deg  RySpringStiffness=0  RySpringStiffnessUnits=N*m/deg  RyDampingCoefficient=0  RyDampingCoefficientUnits=N*m/(deg/s)  RyLowerLimitSpecify=off  RyLowerLimitBound=-90  RyLowerLimitBoundUnits=deg  RyLowerLimitStiffness=1e4  RyLowerLimitStiffnessUnits=N*m/deg  RyLowerLimitDamping=10  RyLowerLimitDampingUnits=N*m/(deg/s)  RyLowerLimitTransitionRegionWidth=0.1  RyLowerLimitTransitionRegionWidthUnits=deg  RyUpperLimitSpecify=off  RyUpperLimitBound=90  RyUpperLimitBoundUnits=deg  RyUpperLimitStiffness=1e4  RyUpperLimitStiffnessUnits=N*m/deg  RyUpperLimitDamping=10  RyUpperLimitDampingUnits=N*m/(deg/s)  RyUpperLimitTransitionRegionWidth=0.1  RyUpperLimitTransitionRegionWidthUnits=deg  RyTorqueActuationMode=NoTorque  RyMotionActuationMode=ComputedMotion  RySensePosition=off  RySenseVelocity=off  RySenseAcceleration=off  RySenseTorqueForce=off  RySenseLowerLimitTorqueForce=off  RySenseUpperLimitTorqueForce=off
      settings: LibrarySourceBlock=|
      | sm_car_4post_lib/Suspension and Steering/Linkage/Linkage L/DoubleWishbone/Universal
      | Rod Upright
  Upper Arm : Subsystem  mask{popup_leftRight=Left, hp_in_f=hp_in_f_ua, hp_in_r=hp_in_r_ua, hp_out=hp_out_ua, ua_mass=ua_mass, clr_ua=clr_ua, opc_ua=opc_ua, radius_ua=radius_ua}
      mask prompts: popup_leftRight "Left/Right"; hp_in_f "Inboard Front [xyz] (m)"; hp_in_r "Inboard Rear [xyz] (m)"; hp_out "Outboard [xyz] (m)"; ua_mass "Mass (kg)"; clr_ua "Color [RGB]"; opc_ua "Opacity (0-1)"; radius_ua "Radius (m)"
      mask init:
      | if(popup_leftRight == 1)
      |     rhs_susp = 1;
      | elseif(popup_leftRight == 2)
      |     rhs_susp = -1;
      | end
      | 
      | rhs_hp = [1 rhs_susp 1];
      | 
      | % Calculate lengths and displacments
      | %%%len_front = norm(hp_in_f-hp_out);
      | %%%len_rear  = norm(hp_in_r-hp_out);
      | %%%dist_f2r  = norm(hp_in_f-hp_in_r);
      | 
      | % Calculate angle between arm-to-chassis attachment axis
      | % and outboard hard point at each chassis attachment point
      | %%%angle_f2r_f2out = sm_math_angle_3hp(hp_in_r, hp_in_f, hp_out);
      | %%%angle_r2f_r2out = sm_math_angle_3hp(hp_in_f, hp_in_r, hp_out);
      mask TypeOptions popup_leftRight: Left | Right
      mask TypeOptions clr_ua: Arm F/clr_solid | Arm R/clr_solid
      mask TypeOptions opc_ua: Arm F/opc_solid | Arm R/opc_solid
      mask TypeOptions radius_ua: Arm F/rad_solid | Arm R/rad_solid
      mask DialogControl cont_ua Prompt: UA
      mask DialogControl cont_vis_ua Prompt: Visualization
  Upright : Subsystem  mask(Upright){popup_leftRight=Left, hp_ua_out=hp_out_ua, hp_la_out=hp_out_la, hp_upr_cg=hp_upr_cg, hp_upr_wc=hp_upr_wc, hp_upr_rod=hp_upr_rod, atoe=atoe, acamber=acamber, upr_mass=upr_mass, whl_init_spd=whl_init_spd_lr(whlind), clr_conn_upr=clr_conn_upr, opc_conn_upr=opc_conn_upr, size_conn_upr=size_conn_upr, clr_upr=clr_upr, opc_upr=opc_upr, radius_upr=radius_upr, clr_stub_axle=clr_stub_axle, opc_stub_axle=opc_stub_axle, radius_stub_axle=radius_stub_axle}
      mask prompts: popup_leftRight "Left/Right"; hp_ua_out "Upper Arm Outboard [xyz] (m)"; hp_la_out "Lower Arm Outboard [xyz] (m)"; hp_upr_cg "Center of Mass [xyz] (m)"; hp_upr_wc "Wheel Center [xyz] (m)"; hp_upr_rod "Track Rod Outboard [xyz] (m)"; atoe "Toe Angle (deg)"; acamber "Camber Angle (deg)"; upr_mass "Upright Mass (kg)"; whl_init_spd "Initial Wheel Speed (rad/s)"
      mask help: Suspension linkage that holds wheel bearing.
      mask init:
      | % Set parameter for mirroring (+y or -y)
      | if(popup_leftRight == 1)
      |     rhs_upr = 1;
      | elseif(popup_leftRight == 2)
      |     rhs_upr = -1;
      | end
      | rhs_hp = [1 rhs_upr 1];
      | 
      | % Additional hardpoint at center of upright
      | % Used as attachment points for axle and steering arm
      | hp_upr_ctr = (hp_ua_out+hp_la_out)/2;
      | 
      | % Calculate lengths and displacments
      | %%%len_upr  = norm(hp_la_out-hp_ua_out);
      | len_axle = norm(hp_upr_wc-hp_upr_ctr);
      | %%%len_sarm = norm(hp_upr_rod-hp_upr_ctr);
      | %%%len_cg   = norm(hp_upr_cg-hp_upr_ctr);
      | 
      | % Get angle between steering arm and axle about axis perpendicular to upright z-axis
      | %%%angle_axle2upr_perp = sm_math_angle_3hp(hp_ua_out,hp_upr_ctr,hp_upr_wc);
      | %%%angle_rod2upr_perp = sm_math_angle_3hp(hp_ua_out,hp_upr_ctr,hp_upr_rod);
      | %%%angle_cg2upr_perp = sm_math_angle_3hp(hp_ua_out,hp_upr_ctr,hp_upr_cg);
      | 
      | % Get vectors for axle, arm, and cg relative to upright center
      | %%%vec_upr2rod = hp_upr_rod-hp_upr_ctr;
      | %%%vec_upr2wc  = hp_upr_wc-hp_upr_ctr;
      | %%%vec_upr2cg  = hp_upr_cg-hp_upr_ctr;
      | 
      | % Get angles to rotate upright back to World orientation
      | % Two rotations in sequence, first about x then about y
      | %%%angle_x = -90+atan2d(hp_ua_out(3)-hp_la_out(3),hp_ua_out(2)-hp_la_out(2));
      | %%%angle_y = acosd(sqrt((hp_ua_out(3)-hp_la_out(3))^2+(hp_ua_out(2)-hp_la_out(2))^2)/len_upr);
      | 
      | % Rotate vectors for axle, arm, and cg relative to upright center by these angles
      | %%%vec_upr2rod_inUpr1 = sm_math_rotbasic(vec_upr2rod',-angle_x,'x');
      | %%%vec_upr2rod_inUpr = sm_math_rotbasic(vec_upr2rod_inUpr1,angle_y,'y');
      | 
      | %%%vec_upr2wc_inUpr1  = sm_math_rotbasic(vec_upr2wc',-angle_x,'x');
      | %%%vec_upr2wc_inUpr = sm_math_rotbasic(vec_upr2wc_inUpr1,angle_y,'y');
      | 
      | %%%vec_upr2cg_inUpr1  = sm_math_rotbasic(vec_upr2cg',-angle_x,'x');
      | %%%vec_upr2cg_inUpr = sm_math_rotbasic(vec_upr2cg_inUpr1,angle_y,'y');
      | 
      | % Get angle to steering arm and to axle about upright axis
      | %%%angle_rod2upraxis = atan2d(vec_upr2rod_inUpr(2),vec_upr2rod_inUpr(1));
      | %%%angle_wc2upraxis  = atan2d(vec_upr2wc_inUpr(2),vec_upr2wc_inUpr(1));
      | %%%angle_cg2upraxis  = atan2d(vec_upr2cg_inUpr(2),vec_upr2cg_inUpr(1));
      mask TypeOptions popup_leftRight: Left | Right
      mask TypeOptions upr_mass:
      | Inertia
      | CG/Mass
      mask TypeOptions whl_init_spd: Revolute/Revolute/VelocityTargetValue
      mask TypeOptions clr_conn_upr: Vis Upright LA/GraphicDiffuseColor | Vis Upright UA/GraphicDiffuseColor | Vis Wheel Center/GraphicDiffuseColor
      mask TypeOptions opc_conn_upr: Vis Upright LA/GraphicOpacity | Vis Upright UA/GraphicOpacity | Vis Wheel Center/GraphicOpacity
      mask TypeOptions clr_upr: Upright/clr_solid | Steering Arm/clr_solid
      mask TypeOptions opc_upr: Upright/opc_solid | Steering Arm/opc_solid
      mask TypeOptions radius_upr: Upright/rad_solid | Steering Arm/rad_solid
      mask TypeOptions clr_stub_axle: Axle/GraphicDiffuseColor
      mask TypeOptions opc_stub_axle: Axle/GraphicOpacity
      mask TypeOptions radius_stub_axle: Axle/CylinderRadius
      mask DialogControl cont_upright Prompt: Upright
      mask DialogControl grp_init Prompt: Initialization
      mask DialogControl cont_vis_upr Prompt: Visualization
      mask DialogControl text_clr_upr Prompt: Color [RGB]
      mask DialogControl text_opc_upr Prompt: Opac. (0-1)
      mask DialogControl text_size_upr Prompt: Size (m)
      mask DialogControl text_conn_upr Prompt: Connections
      mask DialogControl text_upright Prompt: Upright
      mask DialogControl text_stub_axle Prompt: Stub Axle
  Vector Concatenate : Concatenate
  Rack : PMIOPort  Side=Right
  Ref : PMIOPort  Port=2  Side=Right
  Axle : PMIOPort  Port=3  Side=Left
  S : PMIOPort  Port=4  Side=Left
  D : PMIOPort  Port=5  Side=Left
  LAo : PMIOPort  Port=6  Side=Left
  WhlAng : Outport
  wires:
  Vector Concatenate/1 -> WhlAng/1
  PS-Simulink Converter3/1 -> Integrator1/1
  Integrator1/1 -> Vector Concatenate/1  "Caster"
  PS-Simulink Converter4/1 -> Integrator2/1
  Integrator2/1 -> Vector Concatenate/2  "Steer"
  connections:
  Transform Track Rod Inboard/RConn1 -- Spherical Rack Rod/LConn1
  Spherical Rack Rod/RConn1 -- Track Rod/RConn1
  Universal Rod Upright/LConn1 -- Track Rod/LConn1
  Spherical UA Upright/RConn1 -- Upright/RConn2
  Primitive Gimbal/LConn1 -- Transform Ref LAo/RConn1 -- Lower Arm/LConn2
  Revolute LA/RConn1 -- Lower Arm/RConn1
  Spherical UA Upright/LConn1 -- Upper Arm/LConn1
  Primitive Gimbal/RConn1 -- Upright/RConn3
  Lower Arm/LConn1 -- Spherical LA Spring/LConn1
  Revolute LA/LConn1 -- Hardpoints/LConn3
  Revolute UA/RConn1 -- Upper Arm/RConn1
  D/RConn1 -- S/RConn1 -- Shock/RConn1
  Rack/RConn1 -- Transform Track Rod Inboard/LConn1
  Upright/RConn1 -- Universal Rod Upright/RConn1
  Revolute UA/LConn1 -- Hardpoints/LConn1
  Ref/RConn1 -- Transform Sensor/LConn1 -- Hardpoints/RConn1
  Universal HP Spring/LConn1 -- Hardpoints/LConn2
  Shock/LConn1 -- Spherical LA Spring/RConn1
  Upright/LConn1 -- Transform Sensor/RConn1 -- Axle/RConn1
  Universal HP Spring/RConn1 -- Shock/RConn2
  PS-Simulink Converter3/LConn1 -- Transform Sensor/RConn2
  PS-Simulink Converter4/LConn1 -- Transform Sensor/RConn3
  Transform Ref LAo/LConn1 -- LAo/RConn1
